simulink model "MainModel_Working_version_With_AAIR"  (R2020a)
settings: Solver=FixedStepAuto  StartTime=0.0  StopTime=10  FixedStep=1e-3  RelTol=1e-3  EnableMultiTasking=on
undefined symbols (not defined in the file): A0, A3, D0, D1, D10, D11, D12, D13, D2, D3, D4, D5, D6, D7, D8, D9, PTA0, PTA1, PTA2, PTB11, PTB2, PTB23, PTB9, PTC16, PTC17, PTC2, PTC3, PTC4, PTD0, PTD1, PTD2, PTD3
libraries: frdmk64flib x19
(part 1 of 2)
settings Model: SimulationMode=external  ExtModeTrigDuration=5  Creator=prana  LastModifiedBy=prana
settings OptimizationCC: EnhancedBackFolding=on  PassReuseOutputArgsAs=Individual arguments  ZeroExternalMemoryAtStartup=off  ZeroInternalMemoryAtStartup=off  MaxStackSize=64  OptimizeBlockOrder=speed  DifferentSizesBufferReuse=on  OptimizationCustomize=off  EfficientTunableParamExpr=on
settings DebuggingCC: ParameterTunabilityLossMsg=error
settings HardwareCC: ProdBitPerPointer=32  ProdBitPerSizeT=32  ProdBitPerPtrDiffT=32  ProdLargestAtomicInteger=Long  ProdLargestAtomicFloat=Double  ProdWordSize=32  ProdHWDeviceType=ARM Compatible->ARM Cortex
settings SFSimCC: MATLABDynamicMemAlloc=off
settings RTWCC: SystemTargetFile=ert.tlc  HardwareBoard=NXP FRDM-K64F  TemplateMakefile=ert_default_tmf  Toolchain=GNU Tools for ARM Embedded Processors
settings CodeAppCC: ForceParamTrailComments=on  IgnoreCustomStorageClasses=off  OperatorAnnotations=on  SimulinkDataObjDesc=on  SFDataObjDesc=on  InsertBlockDesc=on

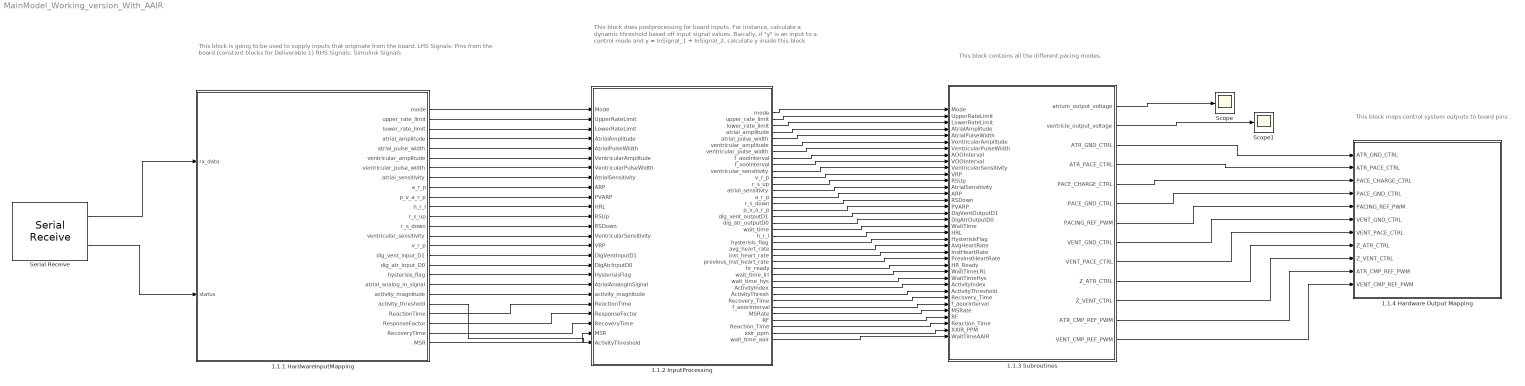
== system MainModel_Working_version_With_AAIR ==
  note: This block does postprocessing for board inputs.
      | For instance, calculate a dynamic threshold based off input signal values.
      | Baically, if "y" is an input to a control mode and y = InSignal_1 + InSignal_2,
      | calculate y inside this block
  note: This block is going to be used to supply inputs that originate from the board.
      | LHS Signals: Pins from the board (constant blocks for Deliverable 1)
      | RHS Signals: Simulink Signals
  note: This block contains all the different pacing modes.
  note: This block maps control system outputs to board pins
  1.1.1 HardwareInputMapping : Subsystem
  1.1.2 InputProcessing : Subsystem
  1.1.3 Subroutines : Subsystem
  1.1.4 Hardware Output Mapping : Subsystem
  Scope : Scope
  Scope1 : Scope
  Serial Receive : frdmk64flib/Serial Receive  SCIModule=0  Baudrate=uint32(9600)  Parity=None  StopBits=1  HardwareFlowControl=None  ByteOrder=LittleEndian  DataType=uint8  DataLength=99  BlockingMode=off  OutputStatus=on  SampleTime=-1
  wires:
  1.1.2 InputProcessing/1(mode) -> 1.1.3 Subroutines/1(Mode)
  1.1.2 InputProcessing/2(upper_rate_limit) -> 1.1.3 Subroutines/2(UpperRateLimit)
  1.1.2 InputProcessing/3(lower_rate_limit) -> 1.1.3 Subroutines/3(LowerRateLimit)
  1.1.2 InputProcessing/4(atrial_amplitude) -> 1.1.3 Subroutines/4(AtrialAmplitude)
  1.1.2 InputProcessing/5(atrial_pulse_width) -> 1.1.3 Subroutines/5(AtrialPulseWidth)
  1.1.2 InputProcessing/6(ventricular_amplitude) -> 1.1.3 Subroutines/6(VentricularAmplitude)
  1.1.2 InputProcessing/7(ventricular_pulse_width) -> 1.1.3 Subroutines/7(VentricularPulseWidth)
  1.1.2 InputProcessing/8(f_aooInterval) -> 1.1.3 Subroutines/8(AOOInterval)
  1.1.2 InputProcessing/9(f_vooInterval) -> 1.1.3 Subroutines/9(VOOInterval)
  1.1.3 Subroutines/1(atrium_output_voltage) -> Scope/1
  1.1.3 Subroutines/2(ventricle_output_voltage) -> Scope1/1
  1.1.1 HardwareInputMapping/1(mode) -> 1.1.2 InputProcessing/1(Mode)
  1.1.1 HardwareInputMapping/2(upper_rate_limit) -> 1.1.2 InputProcessing/2(UpperRateLimit)
  1.1.1 HardwareInputMapping/3(lower_rate_limit) -> 1.1.2 InputProcessing/3(LowerRateLimit)
  1.1.1 HardwareInputMapping/4(atrial_amplitude) -> 1.1.2 InputProcessing/4(AtrialAmplitude)
  1.1.1 HardwareInputMapping/5(atrial_pulse_width) -> 1.1.2 InputProcessing/5(AtrialPulseWidth)
  1.1.1 HardwareInputMapping/6(ventricular_amplitude) -> 1.1.2 InputProcessing/6(VentricularAmplitude)
  1.1.1 HardwareInputMapping/7(ventricular_pulse_width) -> 1.1.2 InputProcessing/7(VentricularPulseWidth)
  1.1.1 HardwareInputMapping/8(atrial_sensitivity) -> 1.1.2 InputProcessing/8(AtrialSensitivity)
  1.1.1 HardwareInputMapping/9(a_r_p) -> 1.1.2 InputProcessing/9(ARP)
  1.1.1 HardwareInputMapping/14(ventricular_sensitivity) -> 1.1.2 InputProcessing/14(VentricularSensitivity)
  1.1.1 HardwareInputMapping/15(v_r_p) -> 1.1.2 InputProcessing/15(VRP)
  1.1.1 HardwareInputMapping/12(r_s_up) -> 1.1.2 InputProcessing/12(RSUp)
  1.1.1 HardwareInputMapping/13(r_s_down) -> 1.1.2 InputProcessing/13(RSDown)
  1.1.1 HardwareInputMapping/10(p_v_a_r_p) -> 1.1.2 InputProcessing/10(PVARP)
  1.1.1 HardwareInputMapping/11(h_r_l) -> 1.1.2 InputProcessing/11(HRL)
  1.1.1 HardwareInputMapping/16(dig_vent_input_D1) -> 1.1.2 InputProcessing/16(DigVentInputD1)
  1.1.1 HardwareInputMapping/17(dig_atr_input_D0) -> 1.1.2 InputProcessing/17(DigAtrInputD0)
  1.1.2 InputProcessing/19(wait_time) -> 1.1.3 Subroutines/19(WaitTime)
  1.1.2 InputProcessing/17(dig_vent_outputD1) -> 1.1.3 Subroutines/17(DigVentOutputD1)
  1.1.2 InputProcessing/18(dig_atr_outputD0) -> 1.1.3 Subroutines/18(DigAtrOutputD0)
  1.1.1 HardwareInputMapping/18(hysterisis_flag) -> 1.1.2 InputProcessing/18(HysterisisFlag)
  1.1.1 HardwareInputMapping/19(atrial_analog_in_signal) -> 1.1.2 InputProcessing/19(AtrialAnalogInSignal)
  1.1.2 InputProcessing/22(avg_heart_rate) -> 1.1.3 Subroutines/22(AvgHeartRate)
  1.1.2 InputProcessing/23(inst_heart_rate) -> 1.1.3 Subroutines/23(InstHeartRate)
  1.1.2 InputProcessing/21(hysterisis_flag) -> 1.1.3 Subroutines/21(HysterisisFlag)
  1.1.2 InputProcessing/11(v_r_p) -> 1.1.3 Subroutines/11(VRP)
  1.1.2 InputProcessing/14(a_r_p) -> 1.1.3 Subroutines/14(ARP)
  1.1.2 InputProcessing/24(previous_inst_heart_rate) -> 1.1.3 Subroutines/24(PrevInstHeartRate)
  1.1.2 InputProcessing/20(h_r_l) -> 1.1.3 Subroutines/20(HRL)
  1.1.3 Subroutines/3(ATR_GND_CTRL) -> 1.1.4 Hardware Output Mapping/1(ATR_GND_CTRL)
  1.1.3 Subroutines/4(ATR_PACE_CTRL) -> 1.1.4 Hardware Output Mapping/2(ATR_PACE_CTRL)
  1.1.3 Subroutines/5(PACE_CHARGE_CTRL) -> 1.1.4 Hardware Output Mapping/3(PACE_CHARGE_CTRL)
  1.1.3 Subroutines/6(PACE_GND_CTRL) -> 1.1.4 Hardware Output Mapping/4(PACE_GND_CTRL)
  1.1.3 Subroutines/7(PACING_REF_PWM) -> 1.1.4 Hardware Output Mapping/5(PACING_REF_PWM)
  1.1.3 Subroutines/8(VENT_GND_CTRL) -> 1.1.4 Hardware Output Mapping/6(VENT_GND_CTRL)
  1.1.3 Subroutines/9(VENT_PACE_CTRL) -> 1.1.4 Hardware Output Mapping/7(VENT_PACE_CTRL)
  1.1.3 Subroutines/10(Z_ATR_CTRL) -> 1.1.4 Hardware Output Mapping/8(Z_ATR_CTRL)
  1.1.3 Subroutines/11(Z_VENT_CTRL) -> 1.1.4 Hardware Output Mapping/9(Z_VENT_CTRL)
  1.1.2 InputProcessing/10(ventricular_sensitivity) -> 1.1.3 Subroutines/10(VentricularSensitivity)
  1.1.2 InputProcessing/13(atrial_sensitivty) -> 1.1.3 Subroutines/13(AtrialSensitivity)
  1.1.3 Subroutines/12(ATR_CMP_REF_PWM) -> 1.1.4 Hardware Output Mapping/10(ATR_CMP_REF_PWM)
  1.1.3 Subroutines/13(VENT_CMP_REF_PWM) -> 1.1.4 Hardware Output Mapping/11(VENT_CMP_REF_PWM)
  1.1.2 InputProcessing/25(hr_ready) -> 1.1.3 Subroutines/25(HR_Ready)
  1.1.2 InputProcessing/16(p_v_a_r_p) -> 1.1.3 Subroutines/16(PVARP)
  1.1.2 InputProcessing/26(wait_time_lrl) -> 1.1.3 Subroutines/26(WaitTimeLRL)
  1.1.2 InputProcessing/27(wait_time_hys) -> 1.1.3 Subroutines/27(WaitTimeHys)
  1.1.2 InputProcessing/15(r_s_down) -> 1.1.3 Subroutines/15(RSDown)
  1.1.2 InputProcessing/12(r_s_up) -> 1.1.3 Subroutines/12(RSUp)
  1.1.1 HardwareInputMapping/20(activity_magnitude) -> 1.1.2 InputProcessing/20(activity_magnitude)
  1.1.2 InputProcessing/28(ActivityIndex) -> 1.1.3 Subroutines/28(ActivityIndex)
  1.1.1 HardwareInputMapping/22(ReactionTime) -> 1.1.2 InputProcessing/21(ReactionTime)
  1.1.1 HardwareInputMapping/23(ResponseFactor) -> 1.1.2 InputProcessing/22(ResponseFactor)
  1.1.1 HardwareInputMapping/24(RecoveryTime) -> 1.1.2 InputProcessing/23(RecoveryTime)
  1.1.1 HardwareInputMapping/25(MSR) -> 1.1.2 InputProcessing/24(MSR)
  1.1.1 HardwareInputMapping/21(activity_threshold) -> 1.1.2 InputProcessing/25(ActivityThreshold)
  1.1.2 InputProcessing/29(ActivityThresh) -> 1.1.3 Subroutines/29(ActivityThreshold)
  1.1.2 InputProcessing/30(Recovery_Time) -> 1.1.3 Subroutines/30(Recovery_Time)
  1.1.2 InputProcessing/31(f_aoorInterval) -> 1.1.3 Subroutines/31(f_aoorInterval)
  1.1.2 InputProcessing/32(MSRate) -> 1.1.3 Subroutines/32(MSRate)
  1.1.2 InputProcessing/33(RF) -> 1.1.3 Subroutines/33(RF)
  1.1.2 InputProcessing/34(Reaction_Time) -> 1.1.3 Subroutines/34(Reaction_Time)
  1.1.2 InputProcessing/35(xxir_ppm) -> 1.1.3 Subroutines/35(XXIR_PPM)
  1.1.2 InputProcessing/36(wait_time_aair) -> 1.1.3 Subroutines/36(WaitTimeAAIR)
  Serial Receive/1 -> 1.1.1 HardwareInputMapping/1(rx_data)
  Serial Receive/2 -> 1.1.1 HardwareInputMapping/2(status)

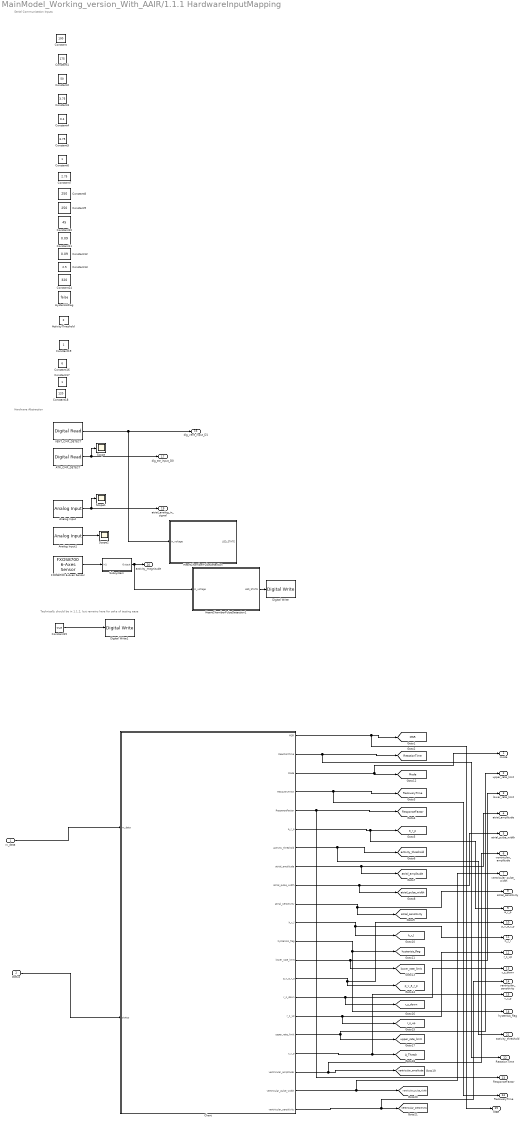
== system MainModel_Working_version_With_AAIR/1.1.1 HardwareInputMapping ==
  note: Technically should be in 1.1.2, but remains here for sake of testing ease
  note: Hardware Abstraction
  note: Serial Communication Inputs
  rx_data : Inport
  status : Inport  Port=2
  ATR_CMP_DETECT : frdmk64flib/Digital Read  Whichpin=PTC16 (D0)  SampleTime=0.001
  ActivityThreshold : Constant  Value=2  OutDataTypeStr=uint32
  Analog Input : frdmk64flib/Analog Input  Whichpin=PTB2 (A0)  SampleTime=0.001
  Analog Input1 : frdmk64flib/Analog Input  Whichpin=PTB11 (A3)  SampleTime=0.001
  Chart : Stateflow chart  TreatAsAtomicUnit=on
  Constant : Constant  Value=100  OutDataTypeStr=uint32
  Constant1 : Constant  Value=175  OutDataTypeStr=uint32
  Constant10 : Constant  Value=45  OutDataTypeStr=uint32
  Constant11 : Constant  Value=0.09  OutDataTypeStr=double
  Constant12 : Constant  Value=0.09  OutDataTypeStr=double
  Constant13 : Constant  Value=2.5  OutDataTypeStr=single
  Constant14 : Constant  Value=320  OutDataTypeStr=uint32
  Constant15 : Constant  Value=true  OutDataTypeStr=boolean
  Constant16 : Constant  Value=6  OutDataTypeStr=uint32
  Constant17 : Constant  OutDataTypeStr=uint32
  Constant18 : Constant  Value=120  OutDataTypeStr=uint32
  Constant19 : Constant  OutDataTypeStr=uint32
  Constant2 : Constant  Value=50  OutDataTypeStr=uint32
  Constant3 : Constant  Value=3.75  OutDataTypeStr=single
  Constant4 : Constant  Value=0.4  OutDataTypeStr=double
  Constant5 : Constant  Value=3.75  OutDataTypeStr=single
  Constant6 : Constant  OutDataTypeStr=double
  Constant7 : Constant  Value=2.75  OutDataTypeStr=single
  Constant8 : Constant  Value=250  OutDataTypeStr=uint32
  Constant9 : Constant  Value=250  OutDataTypeStr=uint32
  Digital Write : frdmk64flib/Digital Write  Whichpin=RED_LED
  Digital Write1 : frdmk64flib/Digital Write  Whichpin=PTD1 (D13)
  FXOS8700 6-Axes Sensor : frdmk64flib/FXOS8700 6-Axes Sensor  Activesensor=Accelerometer only  ODR=800Hz  HybridODR=400Hz  Accelfullrange=-4g to +4g  SampleTime=-1
  HeartChamberPulseDetection : Stateflow chart  TreatAsAtomicUnit=on
  HeartChamberPulseDetection1 : Stateflow chart  TreatAsAtomicUnit=on
  HysterisisFlag : Constant  Value=false  OutDataTypeStr=boolean
  Scope : Scope
  Scope1 : Scope
  Scope2 : Scope
  Subsystem : Subsystem
  VENT_CMP_DETECT : frdmk64flib/Digital Read  Whichpin=PTC17 (D1)  SampleTime=0.001
  mode : Outport
  upper_rate_limit : Outport  Port=2
  lower_rate_limit : Outport  Port=3
  atrial_amplitude : Outport  Port=4
  atrial_pulse_width : Outport  Port=5
  ventricular_amplitude : Outport  Port=6
  ventricular_pulse_width : Outport  Port=7
  atrial_sensitivity : Outport  Port=8
  a_r_p : Outport  Port=9
  p_v_a_r_p : Outport  Port=10
  h_r_l : Outport  Port=11
  r_s_up : Outport  Port=12
  r_s_down : Outport  Port=13
  ventricular_sensitivity : Outport  Port=14
  v_r_p : Outport  Port=15
  dig_vent_input_D1 : Outport  Port=16
  dig_atr_input_D0 : Outport  Port=17
  hysterisis_flag : Outport  Port=18
  atrial_analog_in_signal : Outport  Port=19
  activity_magnitude : Outport  Port=20
  activity_threshold : Outport  Port=21
  ReactionTime : Outport  Port=22
  ResponseFactor : Outport  Port=23
  RecoveryTime : Outport  Port=24
  MSR : Outport  Port=25
  tag scope: A_Thresh=global, MSR=global, Mode=global, ReactionTime=global, RecoveryTime=global, ResponseFactor=global, a_r_p=global, activity_threshold=global, atrial_amplitude=global, atrial_pulse_width=global, atrial_sensitivity=global, h_r_l=global, hysterisis_flag=global, lower_rate_limit=global, p_v_a_r_p=global, r_s_down=global, r_s_up=global, upper_rate_limit=global, ventricular_amplitude=global, ventricular_pulse_width=global, ventricular_sensitivity=global
  wires:
  ATR_CMP_DETECT/1 -> Scope/1, dig_atr_input_D0/1
  Analog Input/1 -> Scope1/1, atrial_analog_in_signal/1
  Constant15/1 -> Digital Write1/1
  Analog Input1/1 -> Scope2/1
  VENT_CMP_DETECT/1 -> dig_vent_input_D1/1, HeartChamberPulseDetection/1(in_voltage)
  HeartChamberPulseDetection1/1(LED_STATE) -> Digital Write/1
  FXOS8700 6-Axes Sensor/1 -> Subsystem/1(In1)
  Subsystem/1(Output) -> HeartChamberPulseDetection1/1(in_voltage), activity_magnitude/1
  Chart/3(Mode) -> [Mode], mode/1
  Chart/1(MSR) -> MSR/1, [MSR]
  Chart/2(ReactionTime) -> ReactionTime/1, [ReactionTime]
  Chart/4(RecoveryTime) -> RecoveryTime/1, [RecoveryTime]
  Chart/5(ResponseFactor) -> ResponseFactor/1, [ResponseFactor]
  Chart/6(a_r_p) -> a_r_p/1, [a_r_p]
  Chart/7(activity_threshold) -> activity_threshold/1, [activity_threshold]
  Chart/8(atrial_amplitude) -> atrial_amplitude/1, [atrial_amplitude]
  Chart/9(atrial_pulse_width) -> atrial_pulse_width/1, [atrial_pulse_width]
  Chart/10(atrial_sensitivity) -> atrial_sensitivity/1, [atrial_sensitivity]
  Chart/11(h_r_l) -> h_r_l/1, [h_r_l]
  Chart/12(hysterisis_flag) -> hysterisis_flag/1, [hysterisis_flag]
  Chart/13(lower_rate_limit) -> [lower_rate_limit], lower_rate_limit/1
  Chart/14(p_v_a_r_p) -> p_v_a_r_p/1, [p_v_a_r_p]
  Chart/15(r_s_down) -> [r_s_down], r_s_down/1
  Chart/16(r_s_up) -> r_s_up/1, [r_s_up]
  Chart/17(upper_rate_limit) -> upper_rate_limit/1, [upper_rate_limit]
  Chart/18(v_r_p) -> v_r_p/1, [A_Thresh]
  Chart/19(ventricular_amplitude) -> ventricular_amplitude/1, [ventricular_amplitude]
  Chart/20(ventricular_pulse_width) -> ventricular_pulse_width/1, [ventricular_pulse_width]
  Chart/21(ventricular_sensitivity) -> ventricular_sensitivity/1, [ventricular_sensitivity]
  rx_data/1 -> Chart/1(rx_data)
  status/1 -> Chart/2(status)

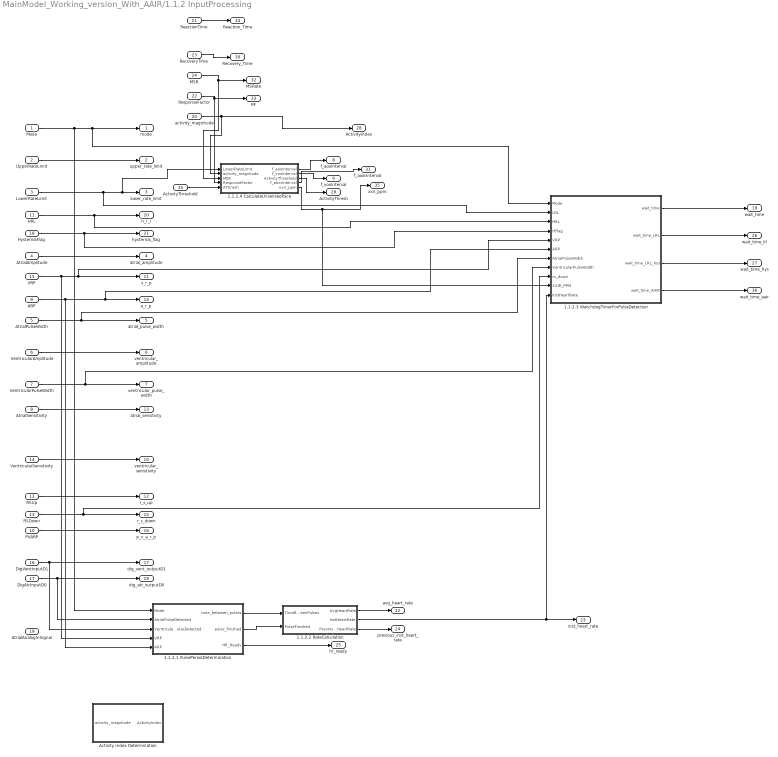
== system MainModel_Working_version_With_AAIR/1.1.2 InputProcessing ==
  Mode : Inport
  UpperRateLimit : Inport  Port=2
  LowerRateLimit : Inport  Port=3
  AtrialAmplitude : Inport  Port=4
  AtrialPulseWidth : Inport  Port=5
  VentricularAmplitude : Inport  Port=6
  VentricularPulseWidth : Inport  Port=7
  AtrialSensitivity : Inport  Port=8
  ARP : Inport  Port=9
  PVARP : Inport  Port=10
  HRL : Inport  Port=11
  RSUp : Inport  Port=12
  RSDown : Inport  Port=13
  VentricularSensitivity : Inport  Port=14
  VRP : Inport  Port=15
  DigVentInputD1 : Inport  Port=16
  DigAtrInputD0 : Inport  Port=17
  HysterisisFlag : Inport  Port=18
  AtrialAnalogInSignal : Inport  Port=19
  activity_magnitude : Inport  Port=20
  ReactionTime : Inport  Port=21
  ResponseFactor : Inport  Port=22
  RecoveryTime : Inport  Port=23
  MSR : Inport  Port=24
  ActivityThreshold : Inport  Port=25
  1.1.2.1 PulsePeriodDetermination : Stateflow chart  TreatAsAtomicUnit=on
  1.1.2.2 RateCalculation : Subsystem
  1.1.2.3 WatchdogTimerForPulseDetection : Stateflow chart  TreatAsAtomicUnit=on
      settings: PortSchema="{\"entries\":[{\"content\":{\"sides\":[{\"content\":{\"connectorIds\":[\"In2\",\"In4\",\"In3\",\"In1\",\"In8\",\"In11\",\"In5\",\"In6\",\"In9\",\"In10\",\"In7\"]},\"type\":\"ConnectorPlacement.EquallySpacedRectSide\",\"uuid\":\"bdcd44c7-b2d4-4456-b1dc-ebe8b4250225\"},{\"content\":{\"connectorIds\":[\"Out1\",\"Out2\",\"Out3\",\"Out4\"],\"side\":\"RIGHT\"},\"type\":\"ConnectorPlacement.EquallySpacedRectSide\",\"uuid\":\"3cd61675-91fc-4dc9-8435-a65c8d2417e3\"},{\"content\":{\"side\":\"TOP\"},\"type\":\"ConnectorPlacement.EquallySpacedRectSide\",\"uuid\":\"27150ff9-b670-45e1-a88f-5aa1ecaf40ee\"}]},\"type\":\"ConnectorPlacement.EquallySpacedConnector\",\"uuid\":\"8013b024-43b4-4f43-9604-3ddd237ba5b0\"}],\"packageUris\":[\"http://schema.mathworks.com/mf0/Connector/R2020b\"],\"version\":\"1.0\"}"
  1.1.2.4 CalculateUnsensedPace : Subsystem
  Activity Index Determination : Stateflow chart  TreatAsAtomicUnit=on
  mode : Outport
  upper_rate_limit : Outport  Port=2
  lower_rate_limit : Outport  Port=3
  atrial_amplitude : Outport  Port=4
  atrial_pulse_width : Outport  Port=5
  ventricular_amplitude : Outport  Port=6
  ventricular_pulse_width : Outport  Port=7
  f_aooInterval : Outport  Port=8
  f_vooInterval : Outport  Port=9
  ventricular_sensitivity : Outport  Port=10
  v_r_p : Outport  Port=11
  r_s_up : Outport  Port=12
  atrial_sensitivty : Outport  Port=13
  a_r_p : Outport  Port=14
  r_s_down : Outport  Port=15
  p_v_a_r_p : Outport  Port=16
  dig_vent_outputD1 : Outport  Port=17
  dig_atr_outputD0 : Outport  Port=18
  wait_time : Outport  Port=19
  h_r_l : Outport  Port=20
  hysterisis_flag : Outport  Port=21
  avg_heart_rate : Outport  Port=22
  inst_heart_rate : Outport  Port=23
  previous_inst_heart_rate : Outport  Port=24
  hr_ready : Outport  Port=25
  wait_time_lrl : Outport  Port=26
  wait_time_hys : Outport  Port=27
  ActivityIndex : Outport  Port=28
  ActivityThresh : Outport  Port=29
  Recovery_Time : Outport  Port=30
  f_aoorInterval : Outport  Port=31
  MSRate : Outport  Port=32
  RF : Outport  Port=33
  Reaction_Time : Outport  Port=34
  xxir_ppm : Outport  Port=35
  wait_time_aair : Outport  Port=36
  wires:
  Mode/1 -> 1.1.2.1 PulsePeriodDetermination/1(Mode), 1.1.2.3 WatchdogTimerForPulseDetection/2(Mode), mode/1
  UpperRateLimit/1 -> upper_rate_limit/1
  LowerRateLimit/1 -> 1.1.2.3 WatchdogTimerForPulseDetection/4(LRL), 1.1.2.4 CalculateUnsensedPace/1(LowerRateLimit), lower_rate_limit/1
  AtrialAmplitude/1 -> atrial_amplitude/1
  AtrialPulseWidth/1 -> 1.1.2.3 WatchdogTimerForPulseDetection/5(AtrialPulseWidth), atrial_pulse_width/1
  VentricularAmplitude/1 -> ventricular_amplitude/1
  VentricularPulseWidth/1 -> 1.1.2.3 WatchdogTimerForPulseDetection/6(VentricularPulseWidth), ventricular_pulse_width/1
  1.1.2.4 CalculateUnsensedPace/1(f_aooInterval) -> f_aooInterval/1
  1.1.2.4 CalculateUnsensedPace/2(f_vooInterval) -> f_vooInterval/1
  VentricularSensitivity/1 -> ventricular_sensitivity/1
  VRP/1 -> 1.1.2.1 PulsePeriodDetermination/4(VRP), 1.1.2.3 WatchdogTimerForPulseDetection/8(VRP), v_r_p/1
  RSUp/1 -> r_s_up/1
  AtrialSensitivity/1 -> atrial_sensitivty/1
  ARP/1 -> 1.1.2.1 PulsePeriodDetermination/5(ARP), 1.1.2.3 WatchdogTimerForPulseDetection/11(ARP), a_r_p/1
  RSDown/1 -> 1.1.2.3 WatchdogTimerForPulseDetection/9(rs_down), r_s_down/1
  PVARP/1 -> p_v_a_r_p/1
  HRL/1 -> 1.1.2.3 WatchdogTimerForPulseDetection/3(HRL), h_r_l/1
  DigVentInputD1/1 -> 1.1.2.1 PulsePeriodDetermination/3(VentricularPulseDetected), dig_vent_outputD1/1
  DigAtrInputD0/1 -> 1.1.2.1 PulsePeriodDetermination/2(AtrialPulseDetected), dig_atr_outputD0/1
  HysterisisFlag/1 -> 1.1.2.3 WatchdogTimerForPulseDetection/1(HFlag), hysterisis_flag/1
  1.1.2.3 WatchdogTimerForPulseDetection/1(wait_time) -> wait_time/1
  1.1.2.1 PulsePeriodDetermination/1(time_between_pulses) -> 1.1.2.2 RateCalculation/1(TimeBetweenPulses)
  1.1.2.2 RateCalculation/1(AvgHeartRate) -> avg_heart_rate/1
  1.1.2.2 RateCalculation/3(PrevInstHeartRate) -> previous_inst_heart_rate/1
  1.1.2.2 RateCalculation/2(InstHeartRate) -> 1.1.2.3 WatchdogTimerForPulseDetection/7(InstHeartRate), inst_heart_rate/1
  1.1.2.1 PulsePeriodDetermination/3(HR_Ready) -> hr_ready/1
  1.1.2.1 PulsePeriodDetermination/2(pulse_finished) -> 1.1.2.2 RateCalculation/2(PulseFinished)
  1.1.2.3 WatchdogTimerForPulseDetection/2(wait_time_LRL) -> wait_time_lrl/1
  1.1.2.3 WatchdogTimerForPulseDetection/3(wait_time_LRL_hys) -> wait_time_hys/1
  activity_magnitude/1 -> 1.1.2.4 CalculateUnsensedPace/2(activity_magnitude), ActivityIndex/1
  ActivityThreshold/1 -> 1.1.2.4 CalculateUnsensedPace/5(AThresh)
  1.1.2.4 CalculateUnsensedPace/3(ActivityThreshold) -> ActivityThresh/1
  MSR/1 -> 1.1.2.4 CalculateUnsensedPace/3(MSR), MSRate/1
  ResponseFactor/1 -> RF/1, 1.1.2.4 CalculateUnsensedPace/4(ResponseFactor)
  RecoveryTime/1 -> Recovery_Time/1
  1.1.2.4 CalculateUnsensedPace/4(f_aoorInterval) -> f_aoorInterval/1
  ReactionTime/1 -> Reaction_Time/1
  1.1.2.4 CalculateUnsensedPace/5(xxir_ppm) -> 1.1.2.3 WatchdogTimerForPulseDetection/10(XXIR_PPM), xxir_ppm/1
  1.1.2.3 WatchdogTimerForPulseDetection/4(wait_time_AAIR) -> wait_time_aair/1

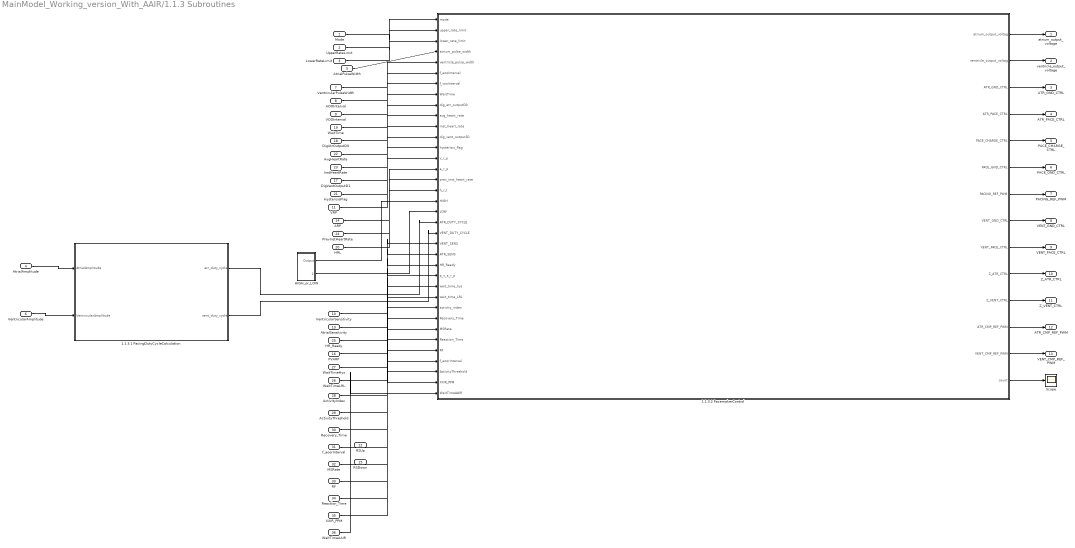
== system MainModel_Working_version_With_AAIR/1.1.3 Subroutines ==
  Mode : Inport
  UpperRateLimit : Inport  Port=2
  LowerRateLimit : Inport  Port=3
  AtrialAmplitude : Inport  Port=4
  AtrialPulseWidth : Inport  Port=5  OutDataTypeStr=double
  VentricularAmplitude : Inport  Port=6
  VentricularPulseWidth : Inport  Port=7  OutDataTypeStr=double
  AOOInterval : Inport  Port=8
  VOOInterval : Inport  Port=9
  VentricularSensitivity : Inport  Port=10
  VRP : Inport  Port=11
  RSUp : Inport  Port=12
  AtrialSensitivity : Inport  Port=13
  ARP : Inport  Port=14
  RSDown : Inport  Port=15
  PVARP : Inport  Port=16
  DigVentOutputD1 : Inport  Port=17
  DigAtrOutputD0 : Inport  Port=18
  WaitTime : Inport  Port=19
  HRL : Inport  Port=20
  HysterisisFlag : Inport  Port=21
  AvgHeartRate : Inport  Port=22
  InstHeartRate : Inport  Port=23
  PrevInstHeartRate : Inport  Port=24
  HR_Ready : Inport  Port=25
  WaitTimeLRL : Inport  Port=26
  WaitTimeHys : Inport  Port=27
  ActivityIndex : Inport  Port=28
  ActivityThreshold : Inport  Port=29
  Recovery_Time : Inport  Port=30
  f_aoorInterval : Inport  Port=31
  MSRate : Inport  Port=32
  RF : Inport  Port=33
  Reaction_Time : Inport  Port=34
  XXIR_PPM : Inport  Port=35
  WaitTimeAAIR : Inport  Port=36
  1.1.3.1 PacingDutyCycleCalculation : Subsystem
  1.1.3.2 PacemakerControl : Stateflow chart  TreatAsAtomicUnit=on
      settings: PortSchema="{\"entries\":[{\"content\":{\"sides\":[{\"content\":{\"connectorIds\":[\"In1\",\"In2\",\"In3\",\"In4\",\"In5\",\"In6\",\"In7\",\"In8\",\"In12\",\"In10\",\"In11\",\"In9\",\"In13\",\"In14\",\"In15\",\"In16\",\"In17\",\"In18\",\"In19\",\"In20\",\"In21\",\"In22\",\"In23\",\"In24\",\"In25\",\"In26\",\"In27\",\"In28\",\"In29\",\"In30\",\"In31\",\"In32\",\"In33\",\"In34\",\"In35\",\"In36\"]},\"type\":\"ConnectorPlacement.EquallySpacedRectSide\",\"uuid\":\"d7a0a1d4-1adb-4f49-9409-b65f2a410999\"},{\"content\":{\"connectorIds\":[\"Out1\",\"Out2\",\"Out3\",\"Out4\",\"Out5\",\"Out6\",\"Out7\",\"Out8\",\"Out9\",\"Out10\",\"Out11\",\"Out12\",\"Out13\",\"Out14\"],\"side\":\"RIGHT\"},\"type\":\"ConnectorPlacement.EquallySpacedRectSide\",\"uuid\":\"f178eaad-70cd-4ec4-a78d-12af1cfbe493\"},{\"content\":{\"side\":\"TOP\"},\"type\":\"ConnectorPlacement.EquallySpacedRectSide\",\"uuid\":\"df2c6513-3872-482b-abe5-5bf3da958119\"}]},\"type\":\"ConnectorPlacement.EquallySpacedConnector\",\"uuid\":\"0d6dffcb-0af9-47c5-9cde-377e88cba9d4\"}],\"packageUris\":[\"http://schema.mathworks.com/mf0/Connector/R2020b\"],\"version\":\"1.0\"}"
  HIGH_or_LOW : Subsystem
      settings: PortSchema="{\"entries\":[{\"content\":{\"sides\":[{\"content\":{},\"type\":\"ConnectorPlacement.EquallySpacedRectSide\",\"uuid\":\"49d8c1b3-c71d-4c5e-9f29-3a8fe0514842\"},{\"content\":{\"side\":\"RIGHT\"},\"type\":\"ConnectorPlacement.EquallySpacedRectSide\",\"uuid\":\"0963f443-37bf-457e-bfcb-1d561403e5a9\"},{\"content\":{\"connectorIds\":[\"Out1\",\"Out2\"],\"side\":\"TOP\"},\"type\":\"ConnectorPlacement.EquallySpacedRectSide\",\"uuid\":\"32b78edd-16d0-4f55-b401-e4c12abc873e\"}]},\"type\":\"ConnectorPlacement.EquallySpacedConnector\",\"uuid\":\"974eb872-d95b-4224-a0e6-f13ce9826807\"}],\"packageUris\":[\"http://schema.mathworks.com/mf0/Connector/R2020b\"],\"version\":\"1.0\"}"
  Scope : Scope
  atrium_output_voltage : Outport
  ventricle_output_voltage : Outport  Port=2
  ATR_GND_CTRL : Outport  Port=3
  ATR_PACE_CTRL : Outport  Port=4
  PACE_CHARGE_CTRL : Outport  Port=5
  PACE_GND_CTRL : Outport  Port=6
  PACING_REF_PWM : Outport  Port=7
  VENT_GND_CTRL : Outport  Port=8
  VENT_PACE_CTRL : Outport  Port=9
  Z_ATR_CTRL : Outport  Port=10
  Z_VENT_CTRL : Outport  Port=11
  ATR_CMP_REF_PWM : Outport  Port=12
  VENT_CMP_REF_PWM : Outport  Port=13
  wires:
  Mode/1 -> 1.1.3.2 PacemakerControl/1(mode)
  1.1.3.2 PacemakerControl/1(atrium_output_voltage) -> atrium_output_voltage/1
  1.1.3.2 PacemakerControl/2(ventricle_output_voltage) -> ventricle_output_voltage/1
  UpperRateLimit/1 -> 1.1.3.2 PacemakerControl/2(upper_rate_limit)
  LowerRateLimit/1 -> 1.1.3.2 PacemakerControl/3(lower_rate_limit)
  AtrialPulseWidth/1 -> 1.1.3.2 PacemakerControl/4(atrium_pulse_width)
  VentricularPulseWidth/1 -> 1.1.3.2 PacemakerControl/5(ventricle_pulse_width)
  AOOInterval/1 -> 1.1.3.2 PacemakerControl/6(f_aooInterval)
  VOOInterval/1 -> 1.1.3.2 PacemakerControl/7(f_vooInterval)
  WaitTime/1 -> 1.1.3.2 PacemakerControl/8(WaitTime)
  DigVentOutputD1/1 -> 1.1.3.2 PacemakerControl/9(dig_vent_outputD1)
  DigAtrOutputD0/1 -> 1.1.3.2 PacemakerControl/12(dig_atr_outputD0)
  AvgHeartRate/1 -> 1.1.3.2 PacemakerControl/10(avg_heart_rate)
  InstHeartRate/1 -> 1.1.3.2 PacemakerControl/11(inst_heart_rate)
  HysterisisFlag/1 -> 1.1.3.2 PacemakerControl/13(hysterisis_flag)
  VRP/1 -> 1.1.3.2 PacemakerControl/14(v_r_p)
  ARP/1 -> 1.1.3.2 PacemakerControl/15(a_r_p)
  PrevInstHeartRate/1 -> 1.1.3.2 PacemakerControl/16(prev_inst_heart_rate)
  HRL/1 -> 1.1.3.2 PacemakerControl/17(h_r_l)
  HIGH_or_LOW/1(Output) -> 1.1.3.2 PacemakerControl/18(HIGH)
  HIGH_or_LOW/2(Output1) -> 1.1.3.2 PacemakerControl/19(LOW)
  1.1.3.2 PacemakerControl/11(Z_VENT_CTRL) -> Z_VENT_CTRL/1
  1.1.3.2 PacemakerControl/10(Z_ATR_CTRL) -> Z_ATR_CTRL/1
  1.1.3.2 PacemakerControl/9(VENT_PACE_CTRL) -> VENT_PACE_CTRL/1
  1.1.3.2 PacemakerControl/8(VENT_GND_CTRL) -> VENT_GND_CTRL/1
  1.1.3.2 PacemakerControl/7(PACING_REF_PWM) -> PACING_REF_PWM/1
  1.1.3.2 PacemakerControl/6(PACE_GND_CTRL) -> PACE_GND_CTRL/1
  1.1.3.2 PacemakerControl/3(ATR_GND_CTRL) -> ATR_GND_CTRL/1
  1.1.3.2 PacemakerControl/4(ATR_PACE_CTRL) -> ATR_PACE_CTRL/1
  1.1.3.2 PacemakerControl/5(PACE_CHARGE_CTRL) -> PACE_CHARGE_CTRL/1
  VentricularSensitivity/1 -> 1.1.3.2 PacemakerControl/22(VENT_SENS)
  AtrialSensitivity/1 -> 1.1.3.2 PacemakerControl/23(ATR_SENS)
  1.1.3.2 PacemakerControl/12(ATR_CMP_REF_PWM) -> ATR_CMP_REF_PWM/1
  1.1.3.2 PacemakerControl/13(VENT_CMP_REF_PWM) -> VENT_CMP_REF_PWM/1
  HR_Ready/1 -> 1.1.3.2 PacemakerControl/24(HR_Ready)
  1.1.3.2 PacemakerControl/14(count) -> Scope/1
  PVARP/1 -> 1.1.3.2 PacemakerControl/25(p_v_a_r_p)
  WaitTimeLRL/1 -> 1.1.3.2 PacemakerControl/27(wait_time_LRL)
  WaitTimeHys/1 -> 1.1.3.2 PacemakerControl/26(wait_time_hys)
  AtrialAmplitude/1 -> 1.1.3.1 PacingDutyCycleCalculation/1(AtrialAmplitude)
  VentricularAmplitude/1 -> 1.1.3.1 PacingDutyCycleCalculation/2(VentricularAmplitude)
  1.1.3.1 PacingDutyCycleCalculation/1(atr_duty_cycle) -> 1.1.3.2 PacemakerControl/20(ATR_DUTY_CYCLE)
  1.1.3.1 PacingDutyCycleCalculation/2(vent_duty_cycle) -> 1.1.3.2 PacemakerControl/21(VENT_DUTY_CYCLE)
  ActivityIndex/1 -> 1.1.3.2 PacemakerControl/28(activity_index)
  ActivityThreshold/1 -> 1.1.3.2 PacemakerControl/34(ActivityThreshold)
  Recovery_Time/1 -> 1.1.3.2 PacemakerControl/29(Recovery_Time)
  f_aoorInterval/1 -> 1.1.3.2 PacemakerControl/33(f_aoorInterval)
  MSRate/1 -> 1.1.3.2 PacemakerControl/30(MSRate)
  RF/1 -> 1.1.3.2 PacemakerControl/32(RF)
  Reaction_Time/1 -> 1.1.3.2 PacemakerControl/31(Reaction_Time)
  XXIR_PPM/1 -> 1.1.3.2 PacemakerControl/35(XXIR_PPM)
  WaitTimeAAIR/1 -> 1.1.3.2 PacemakerControl/36(WaitTimeAAIR)

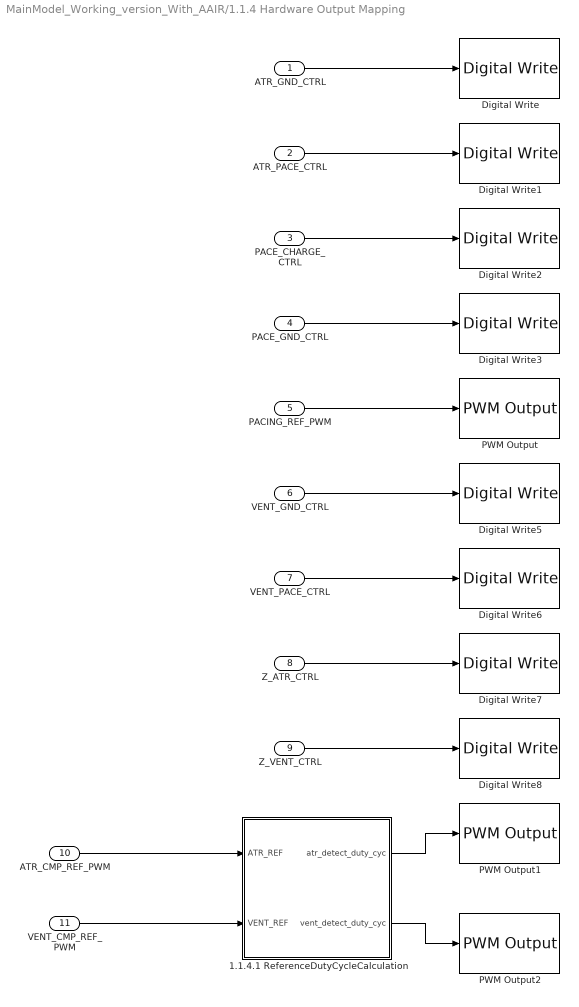
== system MainModel_Working_version_With_AAIR/1.1.4 Hardware Output Mapping ==
  ATR_GND_CTRL : Inport
  ATR_PACE_CTRL : Inport  Port=2
  PACE_CHARGE_CTRL : Inport  Port=3
  PACE_GND_CTRL : Inport  Port=4
  PACING_REF_PWM : Inport  Port=5
  VENT_GND_CTRL : Inport  Port=6
  VENT_PACE_CTRL : Inport  Port=7
  Z_ATR_CTRL : Inport  Port=8
  Z_VENT_CTRL : Inport  Port=9
  ATR_CMP_REF_PWM : Inport  Port=10
  VENT_CMP_REF_PWM : Inport  Port=11
  1.1.4.1 ReferenceDutyCycleCalculation : Subsystem
  Digital Write : frdmk64flib/Digital Write  Whichpin=PTD2 (D11)
  Digital Write1 : frdmk64flib/Digital Write  Whichpin=PTA0 (D8)
  Digital Write2 : frdmk64flib/Digital Write  Whichpin=PTB9 (D2)
  Digital Write3 : frdmk64flib/Digital Write  Whichpin=PTD0 (D10)
  Digital Write5 : frdmk64flib/Digital Write  Whichpin=PTD3 (D12)
  Digital Write6 : frdmk64flib/Digital Write  Whichpin=PTC4 (D9)
  Digital Write7 : frdmk64flib/Digital Write  Whichpin=PTB23 (D4)
  Digital Write8 : frdmk64flib/Digital Write  Whichpin=PTC3 (D7)
  PWM Output : frdmk64flib/PWM Output  Whichpin=PTA2 (D5)  InitialFrequency=2000  InitialDutyCycle=100
  PWM Output1 : frdmk64flib/PWM Output  Whichpin=PTC2 (D6)  InitialFrequency=2000  InitialDutyCycle=20
  PWM Output2 : frdmk64flib/PWM Output  Whichpin=PTA1 (D3)  InitialFrequency=2000  InitialDutyCycle=20
  wires:
  ATR_GND_CTRL/1 -> Digital Write/1
  ATR_PACE_CTRL/1 -> Digital Write1/1
  PACE_CHARGE_CTRL/1 -> Digital Write2/1
  PACE_GND_CTRL/1 -> Digital Write3/1
  VENT_GND_CTRL/1 -> Digital Write5/1
  VENT_PACE_CTRL/1 -> Digital Write6/1
  Z_ATR_CTRL/1 -> Digital Write7/1
  Z_VENT_CTRL/1 -> Digital Write8/1
  PACING_REF_PWM/1 -> PWM Output/1
  ATR_CMP_REF_PWM/1 -> 1.1.4.1 ReferenceDutyCycleCalculation/1(ATR_REF)
  VENT_CMP_REF_PWM/1 -> 1.1.4.1 ReferenceDutyCycleCalculation/2(VENT_REF)
  1.1.4.1 ReferenceDutyCycleCalculation/1(atr_detect_duty_cyc) -> PWM Output1/1
  1.1.4.1 ReferenceDutyCycleCalculation/2(vent_detect_duty_cyc) -> PWM Output2/1

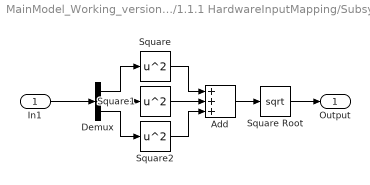
== system MainModel_Working_version_With_AAIR/1.1.1 HardwareInputMapping/Subsystem ==
  In1 : Inport
  Add : Sum  Inputs=+++
  Demux : Demux  Outputs=3
  Square : Math  Operator=square  SaturateOnIntegerOverflow=on
  Square Root : Sqrt  SaturateOnIntegerOverflow=on
  Square1 : Math  Operator=square  SaturateOnIntegerOverflow=on
  Square2 : Math  Operator=square  SaturateOnIntegerOverflow=on
  Output : Outport
  wires:
  Demux/1 -> Square/1
  Demux/2 -> Square1/1
  Demux/3 -> Square2/1
  Square/1 -> Add/1
  Square1/1 -> Add/2
  Square2/1 -> Add/3
  Add/1 -> Square Root/1
  Square Root/1 -> Output/1
  In1/1 -> Demux/1

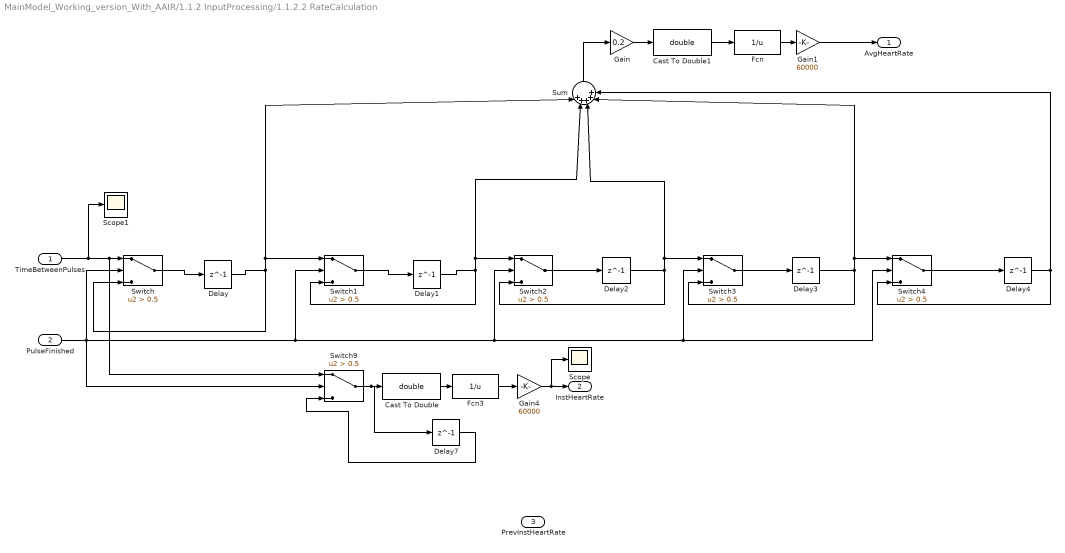
== system MainModel_Working_version_With_AAIR/1.1.2 InputProcessing/1.1.2.2 RateCalculation ==
  TimeBetweenPulses : Inport  OutDataTypeStr=uint32
  PulseFinished : Inport  Port=2  OutDataTypeStr=boolean
  Cast To Double : DataTypeConversion  OutDataTypeStr=double
  Cast To Double1 : DataTypeConversion  OutDataTypeStr=double
  Delay{,1..4} (5 alike) : Delay  DelayLength=1
  Delay7 : Delay  DelayLength=1  InitialCondition=0  SampleTime=0.001
  Fcn : Fcn  Expr=1/u
  Fcn3 : Fcn  Expr=1/u
  Gain : Gain  Gain=0.2
  Gain1 : Gain  Gain=60000
  Gain4 : Gain  Gain=60000
  Scope : Scope
  Scope1 : Scope
  Sum : Sum  Inputs=|+++++
  Switch{,1..4,9} (6 alike) : Switch  Criteria=u2 > Threshold  Threshold=0.5
  AvgHeartRate : Outport  OutDataTypeStr=double
  InstHeartRate : Outport  Port=2  OutDataTypeStr=double
  PrevInstHeartRate : Outport  Port=3  OutDataTypeStr=double
  wires:
  Fcn/1 -> Gain1/1
  Gain4/1 -> Scope/1, InstHeartRate/1
  Fcn3/1 -> Gain4/1
  Switch/1 -> Delay/1
  PulseFinished/1 -> Switch4/2, Switch3/2, Switch2/2, Switch1/2, Switch9/2, Switch/2
  Delay1/1 -> Sum/2, Switch2/1, Switch1/3
  TimeBetweenPulses/1 -> Switch9/1, Switch/1, Scope1/1
  Delay/1 -> Sum/1, Switch1/1, Switch/3
  Sum/1 -> Gain/1
  Switch4/1 -> Delay4/1
  Switch2/1 -> Delay2/1
  Delay2/1 -> Sum/3, Switch3/1, Switch2/3
  Switch3/1 -> Delay3/1
  Delay4/1 -> Sum/5, Switch4/3
  Delay3/1 -> Sum/4, Switch4/1, Switch3/3
  Gain1/1 -> AvgHeartRate/1
  Switch1/1 -> Delay1/1
  Switch9/1 -> Delay7/1, Cast To Double/1
  Delay7/1 -> Switch9/3
  Cast To Double/1 -> Fcn3/1
  Gain/1 -> Cast To Double1/1
  Cast To Double1/1 -> Fcn/1

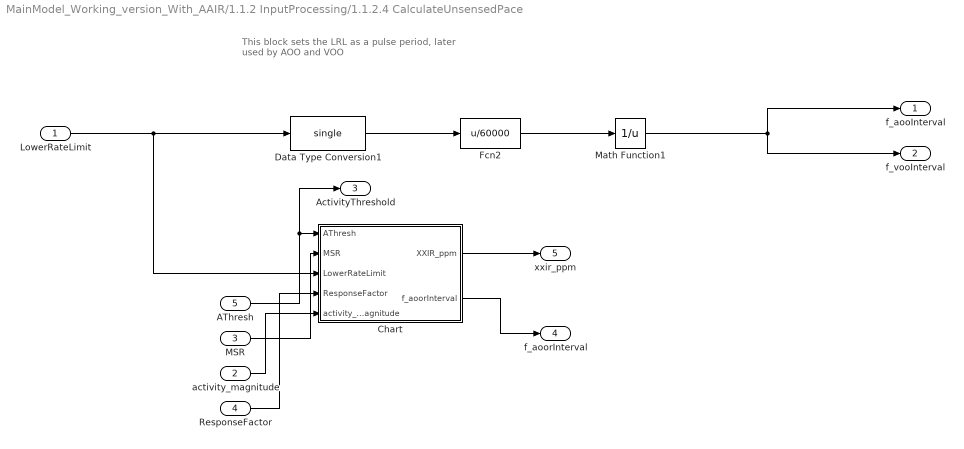
== system MainModel_Working_version_With_AAIR/1.1.2 InputProcessing/1.1.2.4 CalculateUnsensedPace ==
  note: This block sets the LRL as a pulse period, later
      | used by AOO and VOO
  LowerRateLimit : Inport
  activity_magnitude : Inport  Port=2
  MSR : Inport  Port=3
  ResponseFactor : Inport  Port=4
  AThresh : Inport  Port=5
  Chart : Stateflow chart  TreatAsAtomicUnit=on
  Data Type Conversion1 : DataTypeConversion  OutDataTypeStr=single
  Fcn2 : Fcn  Expr=u/60000
  Math Function1 : Math  Operator=reciprocal  SaturateOnIntegerOverflow=on
  f_aooInterval : Outport
  f_vooInterval : Outport  Port=2
  ActivityThreshold : Outport  Port=3
  f_aoorInterval : Outport  Port=4
  xxir_ppm : Outport  Port=5
  wires:
  Math Function1/1 -> f_vooInterval/1, f_aooInterval/1
  Data Type Conversion1/1 -> Fcn2/1
  Fcn2/1 -> Math Function1/1
  LowerRateLimit/1 -> Chart/3(LowerRateLimit), Data Type Conversion1/1
  AThresh/1 -> ActivityThreshold/1, Chart/1(AThresh)
  activity_magnitude/1 -> Chart/5(activity_magnitude)
  Chart/2(f_aoorInterval) -> f_aoorInterval/1
  ResponseFactor/1 -> Chart/4(ResponseFactor)
  MSR/1 -> Chart/2(MSR)
  Chart/1(XXIR_ppm) -> xxir_ppm/1

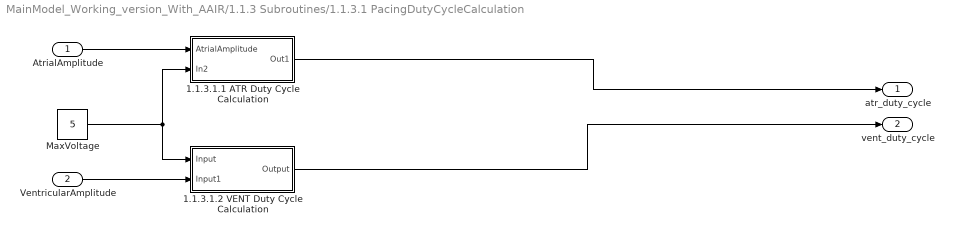
== system MainModel_Working_version_With_AAIR/1.1.3 Subroutines/1.1.3.1 PacingDutyCycleCalculation ==
  AtrialAmplitude : Inport
  VentricularAmplitude : Inport  Port=2
  1.1.3.1.1 ATR Duty Cycle Calculation : Subsystem
  1.1.3.1.2 VENT Duty Cycle Calculation : Subsystem
  MaxVoltage : Constant  Value=5
  atr_duty_cycle : Outport
  vent_duty_cycle : Outport  Port=2
  wires:
  MaxVoltage/1 -> 1.1.3.1.2 VENT Duty Cycle Calculation/1(Input), 1.1.3.1.1 ATR Duty Cycle Calculation/2(In2)
  AtrialAmplitude/1 -> 1.1.3.1.1 ATR Duty Cycle Calculation/1(AtrialAmplitude)
  VentricularAmplitude/1 -> 1.1.3.1.2 VENT Duty Cycle Calculation/2(Input1)
  1.1.3.1.1 ATR Duty Cycle Calculation/1(Out1) -> atr_duty_cycle/1
  1.1.3.1.2 VENT Duty Cycle Calculation/1(Output) -> vent_duty_cycle/1

== system MainModel_Working_version_With_AAIR/1.1.3 Subroutines/HIGH_or_LOW ==
  HIGH : Constant  Value=true
  LOW : Constant  Value=false
  Output : Outport
  Output1 : Outport  Port=2
  wires:
  LOW/1 -> Output1/1
  HIGH/1 -> Output/1

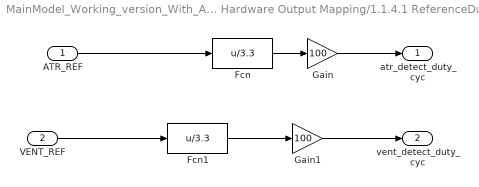
== system MainModel_Working_version_With_AAIR/1.1.4 Hardware Output Mapping/1.1.4.1 ReferenceDutyCycleCalculation ==
  ATR_REF : Inport
  VENT_REF : Inport  Port=2
  Fcn : Fcn  Expr=u/3.3
  Fcn1 : Fcn  Expr=u/3.3
  Gain : Gain  Gain=100
  Gain1 : Gain  Gain=100
  atr_detect_duty_cyc : Outport
  vent_detect_duty_cyc : Outport  Port=2
  wires:
  Fcn/1 -> Gain/1
  VENT_REF/1 -> Fcn1/1
  Gain/1 -> atr_detect_duty_cyc/1
  Fcn1/1 -> Gain1/1
  Gain1/1 -> vent_detect_duty_cyc/1
  ATR_REF/1 -> Fcn/1

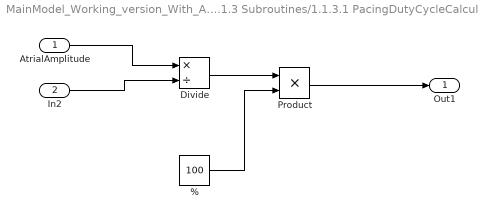
== system MainModel_Working_version_With_AAIR/1.1.3 Subroutines/1.1.3.1 PacingDutyCycleCalculation/1.1.3.1.1 ATR Duty Cycle Calculation ==
  AtrialAmplitude : Inport
  In2 : Inport  Port=2
  % : Constant  Value=100
  Divide : Product  Inputs=*/
  Product : Product
  Out1 : Outport
  wires:
  Divide/1 -> Product/1
  %/1 -> Product/2
  AtrialAmplitude/1 -> Divide/1
  In2/1 -> Divide/2
  Product/1 -> Out1/1

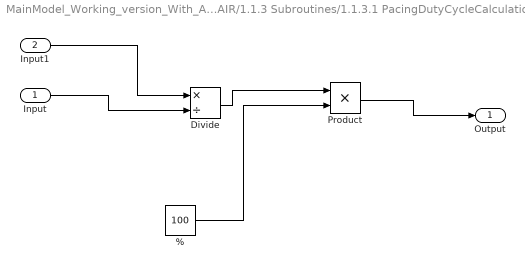
== system MainModel_Working_version_With_AAIR/1.1.3 Subroutines/1.1.3.1 PacingDutyCycleCalculation/1.1.3.1.2 VENT Duty Cycle Calculation ==
  Input : Inport
  Input1 : Inport  Port=2
  % : Constant  Value=100
  Divide : Product  Inputs=*/
  Product : Product
  Output : Outport
  wires:
  Input/1 -> Divide/2
  Input1/1 -> Divide/1
  %/1 -> Product/2
  Divide/1 -> Product/1
  Product/1 -> Output/1

== stateflow chart MainModel_Working_version_With_AAIR/1.1.2 InputProcessing/1.1.2.3 WatchdogTimerForPulseDetection ==
  state HysterisisSelection
    entry:
    time_minute = 60000; % ms/s
    smoothing_rate= InstHeartRate*(1-rs_down);
    total_lower_rate_time = 0;
  state AAI
    entry:
    tot_wait_time = time_minute-((ARP+AtrialPulseWidth)*smoothing_rate);
    wait_time = tot_wait_time / smoothing_rate;
    total_lower_rate_time = time_minute-((ARP+AtrialPulseWidth)*LRL);
    %total_lower_rate_time = time_minute - ((250 + 0.4)*50);
    wait_time_LRL= total_lower_rate_time/ LRL;
    %total_lower_rate_time_hys= time_minute - ((250 + 0.4)*45);
    %wait_time_LRL_hys= total_lower_rate_time_hys/ 45;
    total_lower_rate_time_hys= time_minute - ((ARP + AtrialPulseWidth)*HRL);
    wait_time_LRL_hys= total_lower_rate_time_hys/ HRL;
  state AAIR
    entry:
    tot_wait_time = time_minute-((ARP+AtrialPulseWidth)*smoothing_rate);
    wait_time = tot_wait_time / smoothing_rate;
    total_AAIR_rate_time = time_minute-((ARP+AtrialPulseWidth)*XXIR_PPM);
    wait_time_AAIR= total_AAIR_rate_time/ XXIR_PPM;
    %For LRL so might not need for this mode, but again, left it here for now
    total_lower_rate_time = time_minute-((ARP+AtrialPulseWidth)*LRL);
    wait_time_LRL= total_lower_rate_time/ LRL;
    %For hysterisis so might not be needed for AAIR, but doesn't hurt to leave for now
    total_lower_rate_time_hys= time_minute - ((ARP + AtrialPulseWidth)*HRL);
    wait_time_LRL_hys= total_lower_rate_time_hys/ HRL;
  state VVI
    entry:
    tot_wait_time = time_minute-((VRP+VentricularPulseWidth)*smoothing_rate);
    wait_time = tot_wait_time / smoothing_rate;
    %total_lower_rate_time = time_minute - ((320 + 1)*50);
    total_lower_rate_time = time_minute - ((VRP+VentricularPulseWidth)*LRL);
    wait_time_LRL= total_lower_rate_time/ LRL;
  (default) -> HysterisisSelection
  HysterisisSelection -> VVI [order 2] : [Mode==222]
  HysterisisSelection -> AAI [order 1] : [Mode==112]
  HysterisisSelection -> AAIR [order 3] : [Mode==1121]
  data: HFlag input; Mode input; HRL input; LRL input uint32; AtrialPulseWidth input double; VentricularPulseWidth input double; InstHeartRate input double; VRP input uint32; rs_down input double; XXIR_PPM input; ARP input uint32; wait_time output; tot_wait_time local uint32; time_minute local uint32; smoothing_rate local double; wait_time_LRL output; total_lower_rate_time local uint32; wait_time_LRL_hys output; total_lower_rate_time_hys local; wait_time_AAIR output; total_AAIR_rate_time local

== stateflow chart MainModel_Working_version_With_AAIR/1.1.1 HardwareInputMapping/HeartChamberPulseDetection1 ==
  state default
    entry:
    LED_STATE = false
  state led_on
    entry:
    LED_STATE = true
  (default) -> default
  default -> led_on : [in_voltage < -2 | in_voltage > 2]
  led_on -> default : [in_voltage ~= 0]
  data: LED_STATE output boolean; in_voltage input

== stateflow chart MainModel_Working_version_With_AAIR/1.1.3 Subroutines/1.1.3.2 PacemakerControl ==
  state AAI
    state initializations
      entry:
      ATR_CMP_REF_PWM = ATR_SENS;
      %atrium_output_voltage  = 0;
      count=0;
    state Hysterisis_mode_ON
      entry:
      count = count +1;
    state Hysterisis_mode_OFF
      entry:
      count=count+1;
    state Pulse
      entry:
      %atrium_output_voltage = atrium_pulse_amplitude;
      ATR_PACE_CTRL=LOW;
      VENT_PACE_CTRL=LOW;
      PACING_REF_PWM=ATR_DUTY_CYCLE;
      PACE_CHARGE_CTRL=HIGH;
      PACE_GND_CTRL=HIGH;
      Z_ATR_CTRL=LOW;
      Z_VENT_CTRL=LOW;
      ATR_GND_CTRL=HIGH;
      VENT_GND_CTRL=LOW;
    state CHARGE
      entry:
      %atrium_output_voltage = atrium_pulse_amplitude;
      PACE_CHARGE_CTRL=LOW;
      PACE_GND_CTRL=HIGH;
      ATR_PACE_CTRL=HIGH;
      ATR_GND_CTRL=LOW;
      Z_ATR_CTRL=LOW;
      Z_VENT_CTRL=LOW;
      VENT_GND_CTRL=LOW;
      VENT_PACE_CTRL=LOW;
      PACING_REF_PWM=ATR_DUTY_CYCLE;
      %||((count>WaitTime) && (dig_atr_outputD0 == LOW))
    (default) -> AAI.initializations
    AAI.initializations -> AAI.Hysterisis_mode_ON [order 2] : [hysterisis_flag==1 && after(wait_time_LRL, msec)]
    AAI.initializations -> AAI.Hysterisis_mode_OFF [order 1] : [hysterisis_flag==0 && after(wait_time_LRL, msec)]
    AAI.Pulse -> AAI.initializations : [after(a_r_p,msec)]
    AAI.Hysterisis_mode_ON -> AAI.Hysterisis_mode_ON [order 2] : [(count<=WaitTime)&&(~(dig_atr_outputD0 == LOW && inst_heart_rate<lower_rate_limit))]
    AAI.Hysterisis_mode_OFF -> AAI.Hysterisis_mode_OFF [order 1] : [(count<=WaitTime)&&(~(dig_atr_outputD0 == LOW && inst_heart_rate<lower_rate_limit))]
    AAI.Hysterisis_mode_ON -> AAI.CHARGE [order 1] : [(dig_atr_outputD0 == LOW && inst_heart_rate<h_r_l)]
    AAI.Hysterisis_mode_OFF -> AAI.CHARGE [order 2] : [(dig_atr_outputD0 == LOW && inst_heart_rate<lower_rate_limit)]
    AAI.CHARGE -> AAI.Pulse : [after(atrium_pulse_width,msec)]
  state AOOR
    state CHARGE
      entry:
      ATR_PACE_CTRL=LOW;
      VENT_PACE_CTRL=LOW;
      PACING_REF_PWM=ATR_DUTY_CYCLE;
      PACE_CHARGE_CTRL=HIGH;
      PACE_GND_CTRL=HIGH;
      Z_ATR_CTRL=LOW;
      Z_VENT_CTRL=LOW;
      ATR_GND_CTRL=HIGH;
      VENT_GND_CTRL=LOW;
      %atrium_output_voltage = atrium_pulse_amplitude;
      %exit:
      %atrium_output_voltage = 0;
    state DISCHARGE
      entry:
      PACE_CHARGE_CTRL=LOW;
      PACE_GND_CTRL=HIGH;
      ATR_PACE_CTRL=HIGH;
      ATR_GND_CTRL=LOW;
      Z_ATR_CTRL=LOW;
      Z_VENT_CTRL=LOW;
      VENT_GND_CTRL=LOW;
      VENT_PACE_CTRL=LOW;
      PACING_REF_PWM=ATR_DUTY_CYCLE;
      %atrium_output_voltage = 0;
      %exit:
      %atrium_output_voltage = atrium_pulse_amplitude;
    (default) -> AOOR.CHARGE
    AOOR.DISCHARGE -> AOOR.CHARGE : [[after(f_aoorInterval-atrium_pulse_width,msec) && activity_index < ActivityThreshold]]
    AOOR.CHARGE -> AOOR.DISCHARGE : [[after(atrium_pulse_width,msec)]]
  state AAIR
    state initializations
      entry:
      ATR_CMP_REF_PWM = ATR_SENS;
      %atrium_output_voltage  = 0;
    state Hysterisis_mode_ON
      entry:
    state Hysterisis_mode_OFF
      entry:
    state Pulse
      entry:
      %atrium_output_voltage = atrium_pulse_amplitude;
      ATR_PACE_CTRL=LOW;
      VENT_PACE_CTRL=LOW;
      PACING_REF_PWM=ATR_DUTY_CYCLE;
      PACE_CHARGE_CTRL=HIGH;
      PACE_GND_CTRL=HIGH;
      Z_ATR_CTRL=LOW;
      Z_VENT_CTRL=LOW;
      ATR_GND_CTRL=HIGH;
      VENT_GND_CTRL=LOW;
    state CHARGE
      entry:
      %atrium_output_voltage = atrium_pulse_amplitude;
      PACE_CHARGE_CTRL=LOW;
      PACE_GND_CTRL=HIGH;
      ATR_PACE_CTRL=HIGH;
      ATR_GND_CTRL=LOW;
      Z_ATR_CTRL=LOW;
      Z_VENT_CTRL=LOW;
      VENT_GND_CTRL=LOW;
      VENT_PACE_CTRL=LOW;
      PACING_REF_PWM=ATR_DUTY_CYCLE;
      %||((count>WaitTime) && (dig_atr_outputD0 == LOW))
    (default) -> AAIR.initializations
    AAIR.initializations -> AAIR.Hysterisis_mode_ON [order 2] : [hysterisis_flag==1 && after(WaitTimeAAIR, msec)]
    AAIR.initializations -> AAIR.Hysterisis_mode_OFF [order 1] : [hysterisis_flag==0 && after(WaitTimeAAIR, msec)]
    AAIR.Pulse -> AAIR.initializations : [after(a_r_p,msec)]
    AAIR.Hysterisis_mode_ON -> AAIR.CHARGE : [(dig_atr_outputD0 == LOW  && inst_heart_rate<(XXIR_PPM-5))]
    AAIR.Hysterisis_mode_OFF -> AAIR.CHARGE : [(dig_atr_outputD0 == LOW  && inst_heart_rate<XXIR_PPM)]
    AAIR.CHARGE -> AAIR.Pulse : [after(atrium_pulse_width,msec)]
  state AOO
    state CHARGE
      entry:
      ATR_PACE_CTRL=LOW;
      VENT_PACE_CTRL=LOW;
      PACING_REF_PWM=ATR_DUTY_CYCLE;
      PACE_CHARGE_CTRL=HIGH;
      PACE_GND_CTRL=HIGH;
      Z_ATR_CTRL=LOW;
      Z_VENT_CTRL=LOW;
      ATR_GND_CTRL=HIGH;
      VENT_GND_CTRL=LOW;
      %atrium_output_voltage = atrium_pulse_amplitude;
      %exit:
      %atrium_output_voltage = 0;
    state DISCHARGE
      entry:
      PACE_CHARGE_CTRL=LOW;
      PACE_GND_CTRL=HIGH;
      ATR_PACE_CTRL=HIGH;
      ATR_GND_CTRL=LOW;
      Z_ATR_CTRL=LOW;
      Z_VENT_CTRL=LOW;
      VENT_GND_CTRL=LOW;
      VENT_PACE_CTRL=LOW;
      PACING_REF_PWM=ATR_DUTY_CYCLE;
      %atrium_output_voltage = 0;
      %exit:
      %atrium_output_voltage = atrium_pulse_amplitude;
    (default) -> AOO.CHARGE
    AOO.DISCHARGE -> AOO.CHARGE : [after(atrium_pulse_width,msec)]
    AOO.CHARGE -> AOO.DISCHARGE : [after(f_aooInterval-atrium_pulse_width,msec)]
  state Initialize
    entry:
    AOO = 100;
    VOO = 200;
    AAI = 112;
    VVI = 222;
    AOOR = 1000;
    AAIR = 1120;
    VOOR = 2000;
    VVIR = 2220;
  state Standby
    entry:
    atrium_output_voltage = 0;
    ventricle_output_voltage = 0;
  state VOO
    state CHARGE
      entry:
      ATR_PACE_CTRL=LOW;
      VENT_PACE_CTRL=LOW;
      PACING_REF_PWM=VENT_DUTY_CYCLE;
      PACE_CHARGE_CTRL=HIGH;
      PACE_GND_CTRL=HIGH;
      Z_ATR_CTRL=LOW;
      Z_VENT_CTRL=LOW;
      ATR_GND_CTRL=LOW;
      VENT_GND_CTRL=HIGH;
      %atrium_output_voltage = atrium_pulse_amplitude;
      %exit:
      %atrium_output_voltage = 0;
    state DISCHARGE
      entry:
      PACE_CHARGE_CTRL=LOW;
      PACE_GND_CTRL=HIGH;
      ATR_PACE_CTRL=LOW;
      ATR_GND_CTRL=LOW;
      Z_ATR_CTRL=LOW;
      Z_VENT_CTRL=LOW;
      VENT_GND_CTRL=LOW;
      VENT_PACE_CTRL=HIGH;
      PACING_REF_PWM=VENT_DUTY_CYCLE;
      %ventricle_output_voltage = 0;
      %exit:
      %ventricle_output_voltage = ventricle_pulse_amplitude;
    (default) -> VOO.CHARGE
    VOO.DISCHARGE -> VOO.CHARGE : [after(ventricle_pulse_width,msec)]
    VOO.CHARGE -> VOO.DISCHARGE : [after(f_vooInterval-ventricle_pulse_width,msec)]
  state VVI
    state initializations
      entry:
      VENT_CMP_REF_PWM = VENT_SENS;
      %ventricle_output_voltage  = 0;
      count=0;
    state Hysterisis_mode_OFF
      entry:
      count=count+1
    state Pulse
      entry:
      %ventricle_output_voltage = ventricle_pulse_amplitude;
      ATR_PACE_CTRL=LOW;
      VENT_PACE_CTRL=LOW;
      PACING_REF_PWM=VENT_DUTY_CYCLE;
      PACE_CHARGE_CTRL=HIGH;
      PACE_GND_CTRL=HIGH;
      Z_ATR_CTRL=LOW;
      Z_VENT_CTRL=LOW;
      ATR_GND_CTRL=LOW;
      VENT_GND_CTRL=HIGH;
    state Hysterisis_mode_ON
      entry:
      count = count +1;
    state CHARGE
      entry:
      %ventricle_output_voltage = ventricle_pulse_amplitude;
      PACE_CHARGE_CTRL=LOW;
      PACE_GND_CTRL=HIGH;
      ATR_PACE_CTRL=LOW;
      ATR_GND_CTRL=LOW;
      Z_ATR_CTRL=LOW;
      Z_VENT_CTRL=LOW;
      VENT_GND_CTRL=LOW;
      VENT_PACE_CTRL=HIGH;
      PACING_REF_PWM=VENT_DUTY_CYCLE;
      %||((count>WaitTime) && (dig_vent_outputD1 == LOW))
    (default) -> VVI.initializations
    VVI.initializations -> VVI.Hysterisis_mode_ON [order 2] : [hysterisis_flag==1 && after(wait_time_LRL, msec)]
    VVI.initializations -> VVI.Hysterisis_mode_OFF [order 1] : [hysterisis_flag==0 && after(wait_time_LRL, msec)]
    VVI.Pulse -> VVI.initializations : [after(v_r_p,msec)]
    VVI.Hysterisis_mode_OFF -> VVI.Hysterisis_mode_OFF [order 1] : [(count<=WaitTime)&&(~(dig_vent_outputD1 == LOW && inst_heart_rate<lower_rate_limit))]
    VVI.Hysterisis_mode_ON -> VVI.Hysterisis_mode_ON [order 2] : [(count<=WaitTime)&&(~(dig_vent_outputD1 == LOW && inst_heart_rate<lower_rate_limit))]
    VVI.Hysterisis_mode_OFF -> VVI.CHARGE [order 2] : [(dig_vent_outputD1 == LOW && inst_heart_rate<lower_rate_limit)]
    VVI.Hysterisis_mode_ON -> VVI.CHARGE [order 1] : [(dig_vent_outputD1 == LOW && inst_heart_rate<h_r_l)]
    VVI.CHARGE -> VVI.Pulse : [after(ventricle_pulse_width,msec)]
  AOO -> Standby : [mode ~= AOO]
  Standby -> AOO [order 1] : [mode == AOO]
  AAI -> Standby : [mode ~= AAI]
  Standby -> AAI [order 5] : [mode == AAI]
  AOOR -> Standby : [mode ~= AOOR]
  Standby -> AOOR [order 7] : [mode == AOOR]
  AAIR -> Standby : [mode ~= AAIR]
  Standby -> AAIR [order 2] : [mode == AAIR]
  (default) -> Initialize
  Initialize -> Standby : [HR_Ready == true]
  Standby -> Initialize [order 6] : [HR_Ready == false]
  VOO -> Standby : [mode ~= VOO]
  Standby -> VOO [order 4] : [mode == VOO]
  VVI -> Standby : [mode ~= VVI]
  Standby -> VVI [order 3] : [mode == VVI]
  data: mode input uint32; upper_rate_limit input uint32; lower_rate_limit input uint32; atrium_pulse_width input double; ventricle_pulse_width input double; f_aooInterval input single; f_vooInterval input single; atrium_output_voltage output single; ventricle_output_voltage output single; AAI local uint32; VVI local uint32; VOO local int32; AOO local uint32; WaitTime input; dig_vent_outputD1 input; avg_heart_rate input; inst_heart_rate input; dig_atr_outputD0 input; hysterisis_flag input; v_r_p input; a_r_p input; prev_inst_heart_rate input; h_r_l input; ATR_GND_CTRL output; ATR_PACE_CTRL output; PACE_CHARGE_CTRL output; PACE_GND_CTRL output; PACING_REF_PWM output; VENT_GND_CTRL output; VENT_PACE_CTRL output; Z_ATR_CTRL output; Z_VENT_CTRL output; HIGH input; LOW input; ATR_DUTY_CYCLE input; VENT_DUTY_CYCLE input; ATR_CMP_REF_PWM output; VENT_CMP_REF_PWM output; VENT_SENS input; ATR_SENS input; HR_Ready input boolean; count output; p_v_a_r_p input; wait_time_hys input; wait_time_LRL input; activity_index input; Recovery_Time input; MSRate input; Reaction_Time input; RF input; f_aoorInterval input; AOOR local; VVIR local; VOOR local; AAIR local; VLOW local; VHIGH local; MHIGH local; MED local; LLOW local; HHIGH local; ActivityThreshold input; XXIR_PPM input; WaitTimeAAIR input

== stateflow chart MainModel_Working_version_With_AAIR/1.1.2 InputProcessing/Activity Index Determination ==
  state init
    entry:
    a = activity_magnitude;
  state V_Low
    entry:
    ActivityIndex = 1
  state Low
    entry:
    ActivityIndex = 2
  state Med_Low
    entry:
    ActivityIndex = 3
  state Med
    entry:
    ActivityIndex = 4
  state Med_High
    entry:
    ActivityIndex = 5
  state High
    entry:
    ActivityIndex = 6
  state V_High
    entry:
    ActivityIndex = 7
  (default) -> init
  init -> V_Low [order 1] : [a >= 0 && a < 1]
  init -> High [order 6] : [a >= 5 && a < 6]
  init -> V_High [order 7] : [a >= 6 && a < 7]
  init -> Low [order 2] : [a >= 1 && a < 2]
  init -> Med_High [order 5] : [a >=4 && a < 5]
  init -> Med_Low [order 3] : [a >= 2 && a < 3]
  init -> Med [order 4] : [a >=3 && a < 4]
  data: activity_magnitude input; ActivityIndex output; a local
